simulink model "Commande_Sechoir_Hybride"  (R2025b)
settings: Solver=ode45  StartTime=0.0  StopTime=8000  FixedStep=1  RelTol=1e-3
undefined symbols (not defined in the file or in its folder): Kth, tauth, Tsec0
settings Model: Creator=pc  LastModifiedBy=pc

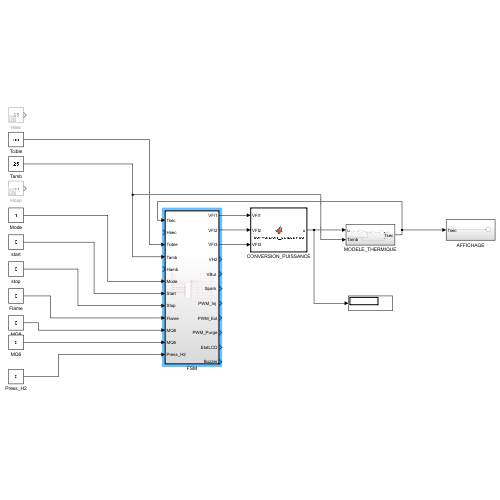
[thumbnail: Simulink's stored preview of the top-level diagram]
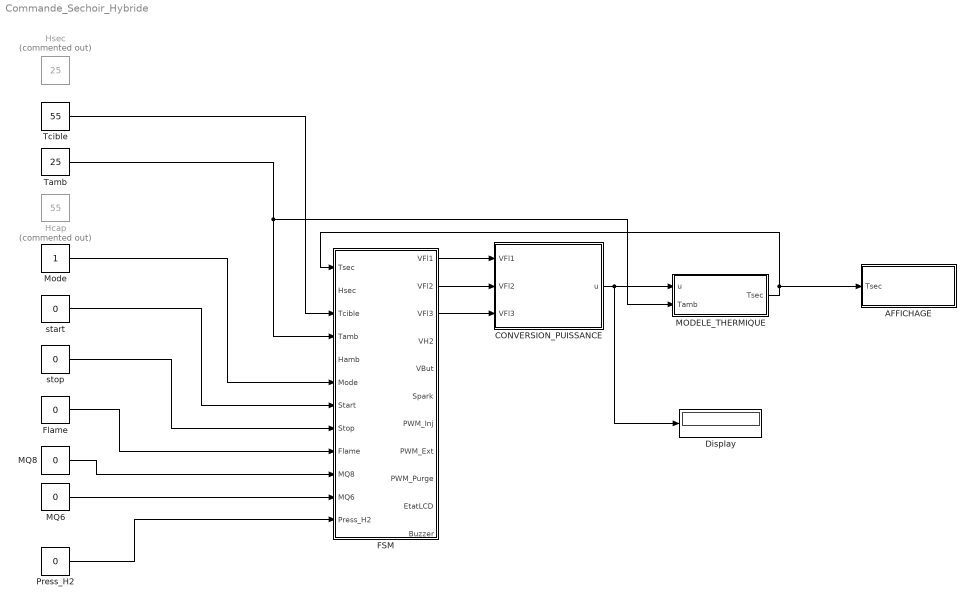
== system Commande_Sechoir_Hybride ==
  AFFICHAGE : Subsystem
  CONVERSION_PUISSANCE : MATLAB Function  TreatAsAtomicUnit=on
  Display : Display
  FSM : Subsystem  TreatAsAtomicUnit=on
  Flame : Constant  Value=0
  Hcap : Constant  Commented=on  Value=55
  Hsec : Constant  Commented=on  Value=25
  MODELE_THERMIQUE : Subsystem
  MQ6 : Constant  Value=0
  MQ8 : Constant  Value=0
  Mode : Constant
  Press_H2 : Constant  Value=0
  Tamb : Constant  Value=25
  Tcible : Constant  Value=55
  start : Constant  Value=0
  stop : Constant  Value=0
  wires:
  FSM/1(VFl1) -> CONVERSION_PUISSANCE/1(VFl1)
  CONVERSION_PUISSANCE/1(u) -> Display/1, MODELE_THERMIQUE/1(u)
  Tamb/1 -> FSM/4("Tamb "), MODELE_THERMIQUE/2(Tamb)
  Tcible/1 -> FSM/3(Tcible)
  Mode/1 -> FSM/6(Mode)
  start/1 -> FSM/7(Start)
  stop/1 -> FSM/8(Stop)
  Flame/1 -> FSM/9("Flame ")
  MQ8/1 -> FSM/10(MQ8)
  MQ6/1 -> FSM/11(MQ6)
  Press_H2/1 -> FSM/12(Press_H2)
  MODELE_THERMIQUE/1(Tsec) -> AFFICHAGE/1(Tsec), FSM/1(Tsec)
  FSM/2(VFl2) -> CONVERSION_PUISSANCE/2(VFl2)
  FSM/3(VFl3) -> CONVERSION_PUISSANCE/3(VFl3)

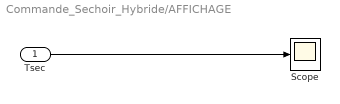
== system Commande_Sechoir_Hybride/AFFICHAGE ==
  Tsec : Inport
  Scope : Scope
  wires:
  Tsec/1 -> Scope/1

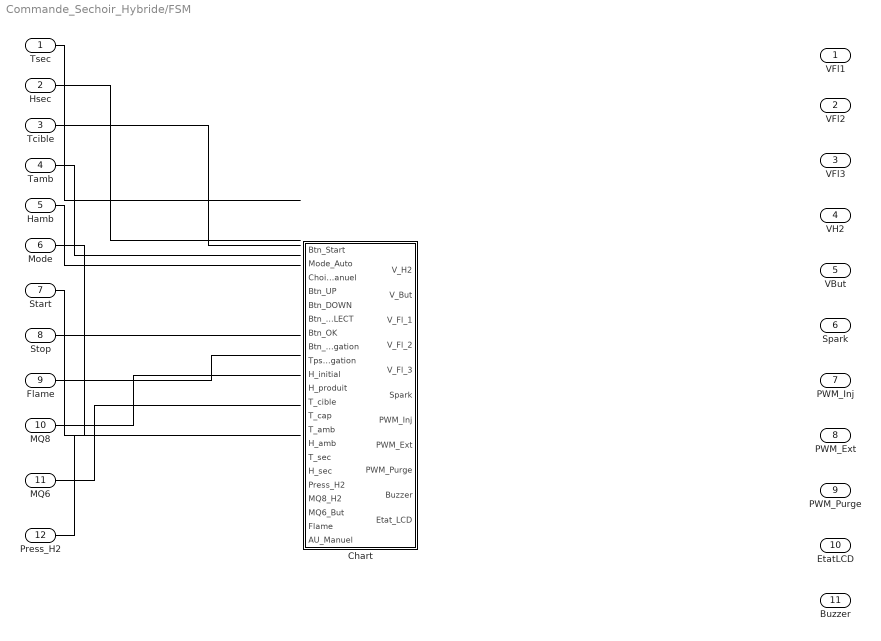
== system Commande_Sechoir_Hybride/FSM ==
  Tsec : Inport
  Hsec : Inport  Port=2
  Tcible : Inport  Port=3
  "Tamb " : Inport  Port=4
  Hamb : Inport  Port=5
  Mode : Inport  Port=6
  Start : Inport  Port=7  OutDataTypeStr=double
  Stop : Inport  Port=8
  "Flame " : Inport  Port=9
  MQ8 : Inport  Port=10
  MQ6 : Inport  Port=11
  Press_H2 : Inport  Port=12
  Chart : Stateflow chart  TreatAsAtomicUnit=on
  VFl1 : Outport
  VFl2 : Outport  Port=2
  VFl3 : Outport  Port=3
  VH2 : Outport  Port=4
  "VBut " : Outport  Port=5
  "Spark " : Outport  Port=6
  "PWM_Inj " : Outport  Port=7
  PWM_Ext : Outport  Port=8
  PWM_Purge : Outport  Port=9
  EtatLCD : Outport  Port=10
  Buzzer : Outport  Port=11
  wires:
  Start/1 -> ?
  Stop/1 -> ?
  "Flame "/1 -> ?
  MQ8/1 -> ?
  MQ6/1 -> ?
  Press_H2/1 -> ?
  Mode/1 -> ?
  "Tamb "/1 -> ?
  Tcible/1 -> ?
  Tsec/1 -> ?
  ? -> VFl1/1
  ? -> VFl2/1
  ? -> VFl3/1
  ? -> VH2/1
  ? -> "VBut "/1
  ? -> "Spark "/1
  ? -> "PWM_Inj "/1
  ? -> PWM_Ext/1
  ? -> PWM_Purge/1
  ? -> EtatLCD/1
  ? -> Buzzer/1
  Hsec/1 -> ?
  Hamb/1 -> ?

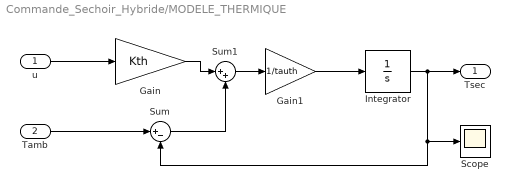
== system Commande_Sechoir_Hybride/MODELE_THERMIQUE ==
  u : Inport
  Tamb : Inport  Port=2
  Gain : Gain  Gain=Kth
  Gain1 : Gain  Gain=1/tauth
  Integrator : Integrator  InitialCondition=Tsec0
  Scope : Scope
      settings: ActiveDisplayYMinimum=16.194004458087669  ActiveDisplayYMaximum=36.797825873537377
  Sum : Sum  Inputs=|+-
  Sum1 : Sum  Inputs=|++
  Tsec : Outport
  wires:
  Tamb/1 -> Sum/1
  u/1 -> Gain/1
  Gain/1 -> Sum1/1
  Sum/1 -> Sum1/2
  Sum1/1 -> Gain1/1
  Gain1/1 -> Integrator/1
  Integrator/1 -> Scope/1, Sum/2, Tsec/1

== stateflow chart Commande_Sechoir_Hybride/FSM/Chart ==
  state FONCTIONNEMENT_NORMAL
    state ATTENTE_DEMARRAGE
    state MODE_SOLAIRE
    state MODE_H2
    state MODE_GPL
    state PROLONGATION
    state FIN_TEMPORISATION
    state SECHAGE_TERMINE
    FONCTIONNEMENT_NORMAL -> ATTENTE_DEMARRAGE [order 1]
    ATTENTE_DEMARRAGE -> MODE_SOLAIRE [order 2] : [Btn_Start == 1 && Mode_Auto == 0 && Choix_Manuel == 1]
    ATTENTE_DEMARRAGE -> MODE_H2 [order 1] : [Btn_Start == 1 && Mode_Auto == 0 && Choix_Manuel == 2]
  state URGENCE_ATEX
  FONCTIONNEMENT_NORMAL -> URGENCE_ATEX [order 1] : [MQ8_H2 >= Seuil_MQ8 || MQ6_But >= Seuil_MQ6 || AU_Manuel == 1]
  data: Btn_Start input uint8 size=[1 1]; Mode_Auto input uint8 size=[1 1]; Choix_Manuel input uint8 size=[1 1]; Btn_UP input uint8 size=[1 1]; Btn_DOWN input uint8 size=[1 1]; Btn_SELECT input uint8 size=[1 1]; Btn_OK input uint8 size=[1 1]; Btn_Prolongation input uint8 size=[1 1]; Tps_Prolongation input double size=[1 1]; H_initial input double size=[1 1] [0..100]; H_produit input double size=[1 1] [0..100]; T_cible input double size=[1 1]; T_cap input double size=[1 1]; T_amb input double size=[1 1]; H_amb input double size=[1 1] [0..100]; T_sec input double size=[1 1]; H_sec input double size=[1 1] [0..100]; Press_H2 input double size=[1 1]; MQ8_H2 input double size=[1 1]; MQ6_But input double size=[1 1]; Flame input uint8 size=[1 1]; AU_Manuel input uint8 size=[1 1]; V_H2 output uint8 size=[1 1] =0; V_But output uint8 size=[1 1] =0; V_Fl_1 output uint8 size=[1 1] =0; V_Fl_2 output uint8 size=[1 1] =0; V_Fl_3 output uint8 size=[1 1] =0; Spark output uint8 size=[1 1] =0; PWM_Inj output uint8 size=[1 1] [0..255] =0; PWM_Ext output uint8 size=[1 1] [0..255] =0; PWM_Purge output uint8 size=[1 1] [0..255] =0; Buzzer output uint8 size=[1 1] =0; Etat_LCD output uint8 size=[1 1] =0; T1_seuil local double size=[1 1] =0; T2_seuil local double size=[1 1] =0; Hhyst local double size=[1 1] =5; H_fin local double size=[1 1] [0..100] =0; chrono_confirmation local double size=[1 1] =0; Temps_Min_Fin local double size=[1 1] =7200

== matlab function Commande_Sechoir_Hybride/CONVERSION_PUISSANCE ==
  data: VFl1 input double; u output; VFl2 input double; VFl3 input double
function u = conversion_puissance(VFl1,VFl2,VFl3)

Pnom = 3000;

if (VFl1 == 1 && VFl2 == 1 && VFl3 == 1)
    u = Pnom;

elseif (VFl1 == 0 && VFl2 == 1 && VFl3 == 1)
    u = 0.67*Pnom;

elseif (VFl1 == 0 && VFl2 == 0 && VFl3 == 1)
    u = 0.33*Pnom;

else
    u = 0;
end
